simulink model "lab1_model4"  (R2021b)
settings: Solver=VariableStepAuto  StartTime=0.0  StopTime=60  RelTol=1e-3
undefined symbols (not defined in the file or in its folder): K_B, K_d, K_d_new
libraries: cstblocks x6
settings Model: Creator=12288  LastModifiedBy=12288

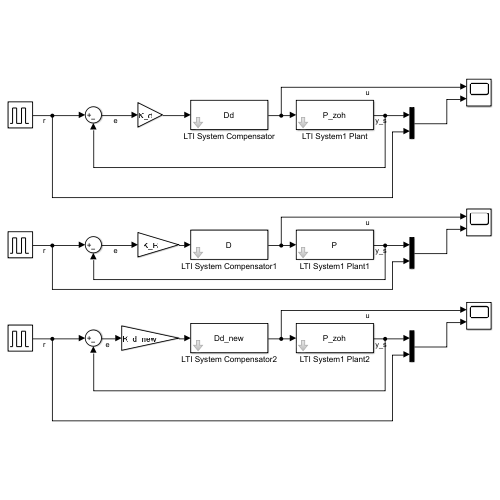
[thumbnail: Simulink's stored preview of the top-level diagram]
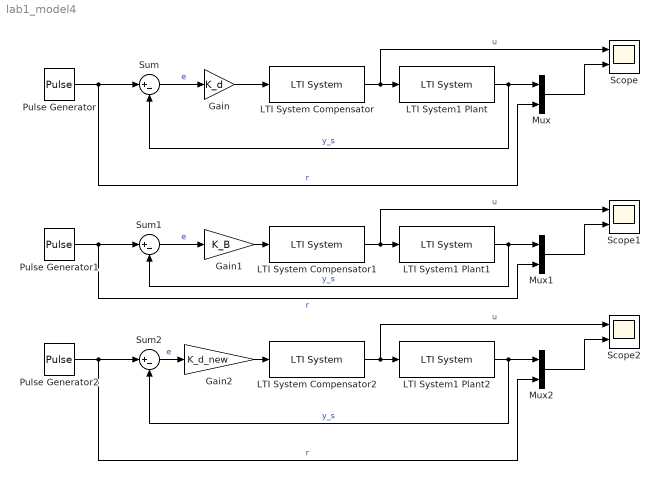
== system lab1_model4 ==
  Gain : Gain  Gain=K_d
  Gain1 : Gain  Gain=K_B
  Gain2 : Gain  Gain=K_d_new
  LTI System Compensator : cstblocks/LTI System  sys=Dd  IC=[]
  LTI System Compensator1 : cstblocks/LTI System  sys=D  IC=[]
  LTI System Compensator2 : cstblocks/LTI System  sys=Dd_new  IC=[]
  LTI System1 Plant : cstblocks/LTI System  sys=P_zoh  IC=[]
  LTI System1 Plant1 : cstblocks/LTI System  sys=P  IC=[]
  LTI System1 Plant2 : cstblocks/LTI System  sys=P_zoh  IC=[]
  Mux : Mux  Inputs=2
  Mux1 : Mux  Inputs=2
  Mux2 : Mux  Inputs=2
  Pulse Generator : DiscretePulseGenerator  PulseType=Time based  Period=10  PulseWidth=50
  Pulse Generator1 : DiscretePulseGenerator  PulseType=Time based  Period=10  PulseWidth=50
  Pulse Generator2 : DiscretePulseGenerator  PulseType=Time based  Period=10  PulseWidth=50
  Scope : Scope  NumInputPorts=2
  Scope1 : Scope  NumInputPorts=2
  Scope2 : Scope  NumInputPorts=2
  Sum : Sum  Inputs=|+-
  Sum1 : Sum  Inputs=|+-
  Sum2 : Sum  Inputs=|+-
  wires:
  Sum/1 -> Gain/1  "e"
  LTI System1 Plant/1 -> Sum/2, Mux/1  "y_s"
  LTI System Compensator/1 -> Scope/1, LTI System1 Plant/1  "u"
  Gain/1 -> LTI System Compensator/1
  Pulse Generator/1 -> Mux/2, Sum/1  "r"
  Mux/1 -> Scope/2
  Sum1/1 -> Gain1/1  "e"
  LTI System Compensator1/1 -> Scope1/1, LTI System1 Plant1/1  "u"
  Pulse Generator1/1 -> Mux1/2, Sum1/1  "r"
  LTI System1 Plant1/1 -> Sum1/2, Mux1/1  "y_s"
  Gain1/1 -> LTI System Compensator1/1
  Mux1/1 -> Scope1/2
  Pulse Generator2/1 -> Mux2/2, Sum2/1  "r"
  Mux2/1 -> Scope2/2
  Sum2/1 -> Gain2/1  "e"
  Gain2/1 -> LTI System Compensator2/1
  LTI System Compensator2/1 -> Scope2/1, LTI System1 Plant2/1  "u"
  LTI System1 Plant2/1 -> Sum2/2, Mux2/1  "y_s"
